simulink library "ddm"  (R2021b)
settings: Solver=VariableStepAuto  StartTime=0.0  StopTime=10.0  RelTol=1e-3
undefined symbols (not defined in the file): ADDM_FrTMTqDev_X_Nm, ADDM_RrTMTqDev_X_Nm, ENUM_ADASACCSTA_ERROR, ENUM_ADASACCSTA_OFF, ENUM_ADASACCSTA_STANDBY, ENUM_ALLOWMOV_ALLOWREADY, ENUM_APS, ENUM_BRKSTA_ERROR, ENUM_BRKSTA_OFF, ENUM_BRKSTA_ON, ENUM_BRKSW_INVALID, ENUM_BRKSW_OFF, ENUM_BRKSW_ON, ENUM_CHGPREACTERRSTA_OBCPRE, ENUM_DCDCFAULTSTA_ANYFAULTLV1, ENUM_DCDCFAULTSTA_ANYFAULTLV2, ENUM_DRIVETRAIN_AWD, ENUM_DRIVETRAIN_FWD, ENUM_DRIVETRAIN_RWD, ENUM_EDUDRTSTA_NORMAL, ENUM_EPBERROR_FAILED, ENUM_EPBSTA_APPLIED, ENUM_EPBSTA_RELEASED, ENUM_ESCAPSSta_APSUNAVAILABLE, ENUM_GEARACTUALPOSN_INVALID, ENUM_GEARACTUALPOSN_P, ENUM_HVBATTREADYPRE_READY, ENUM_HWRESETSTA_HWRESETING, ENUM_MCUWARN_LV0, ENUM_MCUWARN_LV1, ENUM_MCUWARN_LV2, ENUM_MCUWARN_LV3, ENUM_MCUWARN_NOERROR, ENUM_OBCFAULTSTA_ANYFAULT, ENUM_PAS_R2F2, ENUM_PDFAULT_BATTPDFAIL, ENUM_PDFAULT_DCDCDISABLE, ENUM_PDFAULT_MCUDISABLE, ENUM_PDFAULT_MCUDISCHRG, ENUM_POWERSTA_OFF, ENUM_POWERSTA_ON, ENUM_POWERSTA_READY, ENUM_POWERSTA_STANDBY, ENUM_PRESSINDI_LOW, ENUM_PUFAULT_BATTUPFAIL, ENUM_PUFAULT_DCDCENABLEFAIL, ENUM_PUFAULT_PRECHRGCHKFAIL, ENUM_PUFAULT_SAFETYCHKFAIL, ENUM_PWRSTASW_OFF, ENUM_PWRSTASW_OFFA, ENUM_PWRSTASW_OFFCHVCHRG, ENUM_PWRSTASW_OFFCLVCHRG, ENUM_PWRSTASW_ON, ENUM_PWRSTASW_ONHVCHRG, ENUM_PWRSTASW_READY, ENUM_PWRSTASW_STANDBY, ENUM_RAPSErrWarnSta_NORMAL, ENUM_RAPSErrWarnSta_RAPSERRLV1, ENUM_SHIFTCOMMAND_P, ENUM_SHIFTERERRSTA_PBUTTONFAILURE ... (+471)
libraries: hcu_lib x540, simulink x3
(part 15 of 26)

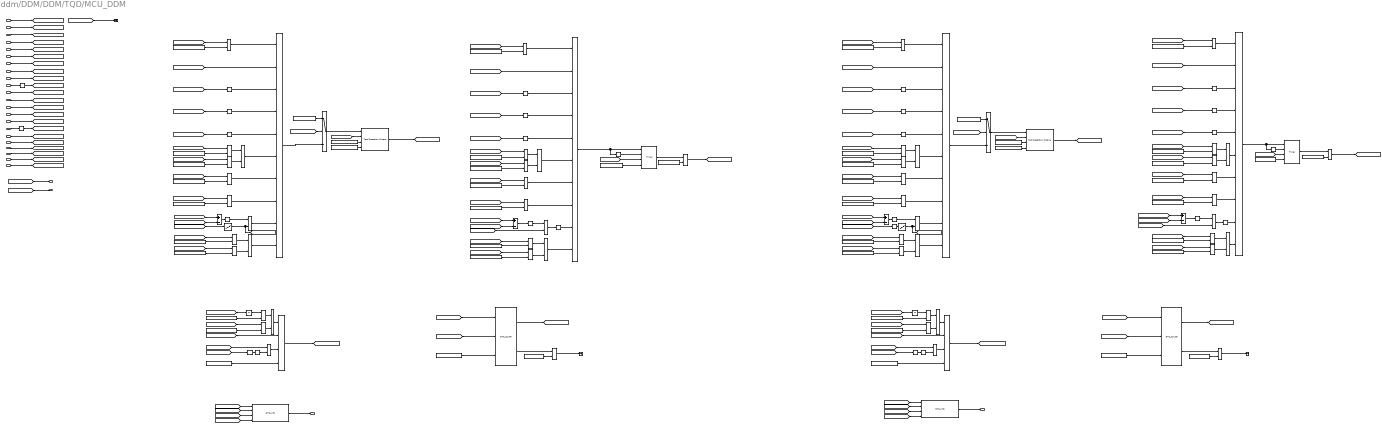
== system ddm/DDM/DDM/TQD/MCU_DDM ==
  note: VINP_FrEDUDrtSta_flg
  note: Front Motor Torque Response Error (FrMCUTqErr)
  note: Test Pass Creteria
  note: Test Dtection Criteria
  note: Test Pass Creteria
  note: Rear Motor Torque Response Error (RrMCUTqErr)
  note: Test Dtection Criteria
  note: Diagnostics and Fault Handling
  note: Release Condition After Decision
  note: Release Condition After Decision
  note: Diagnostics and Fault Handling
  task_time_s : Inport
  VPMM_SysPwrSta_enum : Inport  Port=2
  No_CAN3_BUS_OFF : Inport  Port=3
  VDDM_MCUF1NoComCFS_flg : Inport  Port=4
  VDDM_MCUF1RCErrCFS_flg : Inport  Port=5
  VDDM_MCUF1CSErrCFS_flg : Inport  Port=6
  VINP_VehSpeed_kph : Inport  Port=7
  VINP_FrEDUDrtSta_flg : Inport  Port=8
  VINP_FrEDURealTMTq_Nm : Inport  Port=9
  VTQR_FrTMTqReq_Nm : Inport  Port=10
  VDDM_MCUR1NoComCFS_flg : Inport  Port=11
  VDDM_MCUR1RCErrCFS_flg : Inport  Port=12
  VDDM_MCUR1CSErrCFS_flg : Inport  Port=13
  VINP_RrEDUDrtSta_flg : Inport  Port=14
  VINP_RrEDURealTMTq_Nm : Inport  Port=15
  VTQR_RrTMTqReq_Nm : Inport  Port=16
  VINP_MCUWarnF_enum : Inport  Port=17
  VINP_MCUWarnR_enum : Inport  Port=18
  DTC_clear_request : Inport  Port=19
  VPMM_DrivetrainSelect_enum : Inport  Port=20
  VTQR_FrTqZeroTrans_enum : Inport  Port=21
  VTQR_RrTqZeroTrans_enum : Inport  Port=22
  Abs{,1..3,6} (5 alike) : Abs
  Add{,1..3} (4 alike) : Sum  Inputs=+-
  Constant1 : Constant  Value=ENUM_DRIVETRAIN_FWD
  Constant{3,7,10,31} (4 alike) : Constant  Value=ENUM_TQZEROTRANS_NOZEROTRANS
  Constant{4,11,16,32} (4 alike) : Constant  Value=ENUM_MCUWARN_LV0
  Constant12 : Constant  Value=ENUM_PWRSTASW_STANDBY
  Constant{13,17,19,23,33,44} (6 alike) : Constant  Value=ENUM_PWRSTASW_OFF
  Constant{5,14,21,34} (4 alike) : Constant  Value=ENUM_MCUWARN_NOERROR
  Constant15 : Constant  Value=ENUM_DRIVETRAIN_FWD
  Constant18 : Constant  Value=KDDM_RrMCUTqErrDTC_cnt
  Constant2 : Constant  Value=ENUM_DRIVETRAIN_RWD
  Constant{8,20,26,49} (4 alike) : Constant  Value=ENUM_DRIVETRAIN_AWD
  Constant22 : Constant  Value=ENUM_PWRSTASW_STANDBY
  Constant24 : Constant  Value=FALSE
  Constant{6,25,35,41} (4 alike) : Constant  Value=ENUM_EDUDRTSTA_NORMAL
  Constant28 : Constant  Value=KDDM_RrMCUTqErrDTC_cnt
  Constant29 : Constant  Value=KDDM_TQDDiagnosisOffSW_flg
  Constant30 : Constant  Value=ZERO_INT
  Constant36 : Constant  Value=KDDM_RrMCUTqErrPassTO_s
  Constant37 : Constant  Value=KDDM_RrMCUTqErrDetTO_s
  Constant39 : Constant  Value=KDDM_RrMCUTqErrPassTO_s
  Constant42 : Constant  Value=FALSE
  Constant43 : Constant  Value=KDDM_FrMCUTqErrDTC_cnt
  Constant45 : Constant  Value=KDDM_FrMCUTqErrPassTO_s
  Constant46 : Constant  Value=KDDM_FrMCUTqErrDetTO_s
  Constant51 : Constant  Value=KDDM_TQDDiagnosisOffSW_flg
  Constant52 : Constant  Value=ZERO_INT
  Constant54 : Constant  Value=KDDM_FrMCUTqErrDTC_cnt
  Constant70 : Constant  Value=KDDM_FrMCUTqErrPassTO_s
  Constant9 : Constant  Value=ENUM_DRIVETRAIN_RWD
  DTC_Couter1 : hcu_lib/Basic_Blocks/DTC_Couter
  DTC_Couter3 : hcu_lib/Basic_Blocks/DTC_Couter
  DTC_Info : hcu_lib/Basic_Blocks/DTC_Info
  DTC_Info1 : hcu_lib/Basic_Blocks/DTC_Info
  Delay1 : Delay  DelayLength=1
  Delay2 : Delay  DelayLength=1
  Equal{,1..4,6..7,9..11,14..15,17,20..23,25,28..37} (28 alike) : RelationalOperator  Operator===  OutDataTypeStr=boolean  RndMeth=Simplest
  Equal{5,8,12..13,18,27} (6 alike) : RelationalOperator  OutDataTypeStr=boolean  RndMeth=Simplest
  Equal{16,19,24,26} (4 alike) : RelationalOperator  Operator=~=  OutDataTypeStr=boolean  RndMeth=Simplest
  Logical Operator{1..2,4,16} (4 alike) : Logic  Operator=OR  AllPortsSameDT=off  OutDataTypeStr=boolean
  Logical Operator{3,5,7..10,12..15,17..18,28,34..35,37} (16 alike) : Logic  Operator=NOT  AllPortsSameDT=off  OutDataTypeStr=boolean
  Logical Operator{6,11,27,30} (4 alike) : Logic  Inputs=10  AllPortsSameDT=off  OutDataTypeStr=boolean
  Logical Operator19 : Logic  Operator=OR  Inputs=4  AllPortsSameDT=off  OutDataTypeStr=boolean
  Logical Operator{20..22,43} (4 alike) : Logic  AllPortsSameDT=off  OutDataTypeStr=boolean
  Logical Operator41 : Logic  Operator=OR  Inputs=4  AllPortsSameDT=off  OutDataTypeStr=boolean
  MDDM_FrTMTqDev_Y_Nm : Lookup_n-D  NumberOfTableDimensions=1  BreakpointsForDimension1=ADDM_FrTMTqDev_X_Nm  Table=MDDM_FrTMTqDev_Y_Nm  InternalRulePriority=Speed  RndMeth=Simplest  InputSameDT=on
  MDDM_RrTMTqDev_Y_Nm : Lookup_n-D  NumberOfTableDimensions=1  BreakpointsForDimension1=ADDM_RrTMTqDev_X_Nm  Table=MDDM_RrTMTqDev_Y_Nm  InternalRulePriority=Speed  RndMeth=Simplest  InputSameDT=on
  NOT1 : Logic  Operator=NOT  AllPortsSameDT=off  OutDataTypeStr=boolean
  NOT2 : Logic  Operator=NOT  AllPortsSameDT=off  OutDataTypeStr=boolean
  OR{,1..3} (4 alike) : Logic  Operator=OR  AllPortsSameDT=off  OutDataTypeStr=boolean
  Relational Operator1 : RelationalOperator  Operator=>  OutDataTypeStr=boolean  RndMeth=Simplest
  Relational Operator2 : RelationalOperator  Operator=>  OutDataTypeStr=boolean  RndMeth=Simplest
  Round : Rounding  Operator=round
  Round1 : Rounding  Operator=round
  Switch1 : Switch  Criteria=u2 ~= 0
  Switch6 : Switch  Criteria=u2 ~= 0
  Terminator : Terminator
  Terminator1 : Terminator
  Terminator2 : Terminator
  Test Detection Criteria1 : hcu_lib/Basic_Blocks/Test Detection Criteria
  Test Detection Criteria2 : hcu_lib/Basic_Blocks/Test Detection Criteria
  Timer1 : hcu_lib/Basic_Blocks/Timer
  Timer2 : hcu_lib/Basic_Blocks/Timer
  Unit Delay1 : UnitDelay  SampleTime=-1  HasFrameUpgradeWarning=on
  Unit Delay5 : UnitDelay  SampleTime=-1  HasFrameUpgradeWarning=on
  VDDM_FrMCUTqErrDTC_raw32 : Outport
  VDDM_RrMCUTqErrDTC_raw32 : Outport  Port=2
  VDDM_FrMCUTqErrCFS_flg : Outport  Port=3
  VDDM_RrMCUTqErrCFS_flg : Outport  Port=4
  wires:
  Equal26/1 -> Logical Operator30/1
  Constant44/1 -> Equal26/2
  [VPMM_SysPwrSta_enum] -> Equal26/1
  [No_CAN_BUS_OFF] -> Logical Operator30/2
  Constant4/1 -> Equal6/2
  Constant5/1 -> Equal7/2
  Equal6/1 -> Logical Operator1/1
  Equal7/1 -> Logical Operator1/2
  Logical Operator1/1 -> Logical Operator30/6
  [VINP_FrEDUDrtSta_flg] -> Equal10/1
  Constant6/1 -> Equal10/2
  Equal10/1 -> Logical Operator30/7
  Equal2/1 -> Logical Operator30/8
  [VDDM_MCUF1CSErrCFS_flg] -> Logical Operator10/1
  [VDDM_MCUF1RCErrCFS_flg] -> Logical Operator9/1
  Logical Operator9/1 -> Logical Operator30/4
  [VDDM_MCUF1NoComCFS_flg] -> Logical Operator7/1
  Logical Operator7/1 -> Logical Operator30/3
  Logical Operator10/1 -> Logical Operator30/5
  [VDDM_MCUR1CSErrCFS_flg] -> Logical Operator17/1
  Equal33/1 -> Logical Operator16/1
  [VINP_MCUWarnR_enum] -> Equal33/1
  [VINP_MCUWarnR_enum] -> Equal34/1
  Logical Operator17/1 -> Logical Operator27/5
  Equal34/1 -> Logical Operator16/2
  [VDDM_MCUR1NoComCFS_flg] -> Logical Operator35/1
  Constant33/1 -> Equal24/2
  Equal23/1 -> Logical Operator27/8
  Equal9/1 -> Logical Operator27/7
  [VDDM_MCUR1RCErrCFS_flg] -> Logical Operator37/1
  Constant35/1 -> Equal9/2
  Logical Operator35/1 -> Logical Operator27/3
  Constant32/1 -> Equal33/2
  [VINP_RrEDUDrtSta_flg] -> Equal9/1
  Constant34/1 -> Equal34/2
  [No_CAN_BUS_OFF] -> Logical Operator27/2
  Logical Operator16/1 -> Logical Operator27/6
  Equal24/1 -> Logical Operator27/1
  [VPMM_SysPwrSta_enum] -> Equal24/1
  Logical Operator37/1 -> Logical Operator27/4
  Logical Operator11/1 -> Logical Operator34/1, Timer1/1
  [task_time_s] -> Test Detection Criteria1/2
  [task_time_s] -> Timer1/3
  Constant42/1 -> Switch6/1
  Test Detection Criteria1/1 -> [VDDM_FrMCUTqErrDet_flg]  "VDDM_FrMCUTqErrDet_flg"
  Logical Operator34/1 -> Timer1/2
  Timer1/1 -> Equal27/1
  Constant43/1 -> Test Detection Criteria1/3
  Switch6/1 -> Test Detection Criteria1/1
  Equal27/1 -> [VDDM_FrMCUTqErrPass_flg]  "VDDM_FrMCUTqErrPass_flg"
  Logical Operator30/1 -> Switch6/3
  Constant46/1 -> Test Detection Criteria1/4
  Constant70/1 -> Timer1/4
  Constant45/1 -> Equal27/2
  [VDDM_FrMCUTqErrCFSRls_flg] -> Switch6/2
  [VDDM_FrMCUTqErrDet_flg] -> DTC_Info/1
  DTC_Info/1 -> VDDM_FrMCUTqErrDTC_raw32/1  "VDDM_FrMCUTqErrDTC_raw32"
  [DTC_clear_request] -> DTC_Info/4
  [VDDM_FrMCUTqErrCFS_flg] -> DTC_Info/3
  [VDDM_FrMCUTqErrPass_flg] -> DTC_Info/2
  [VDDM_RrMCUTqErrCFSRls_flg] -> Switch1/2
  Test Detection Criteria2/1 -> [VDDM_RrMCUTqErrDet_flg]  "VDDM_RrMCUTqErrDet_flg"
  [VDDM_RrMCUTqErrDet_flg] -> DTC_Info1/1
  DTC_Info1/1 -> VDDM_RrMCUTqErrDTC_raw32/1  "VDDM_RrMCUTqErrDTC_raw32"
  [DTC_clear_request] -> DTC_Info1/4
  Equal5/1 -> [VDDM_RrMCUTqErrPass_flg]  "VDDM_RrMCUTqErrPass_flg"
  [VDDM_RrMCUTqErrCFS_flg] -> DTC_Info1/3
  Constant39/1 -> Timer2/4
  Constant24/1 -> Switch1/1
  [task_time_s] -> Timer2/3
  Timer2/1 -> Equal5/1
  [VDDM_RrMCUTqErrPass_flg] -> DTC_Info1/2
  [task_time_s] -> Test Detection Criteria2/2
  Constant28/1 -> Test Detection Criteria2/3
  Logical Operator27/1 -> Switch1/3
  Constant37/1 -> Test Detection Criteria2/4
  Switch1/1 -> Test Detection Criteria2/1
  Logical Operator28/1 -> Timer2/2
  Constant36/1 -> Equal5/2
  Logical Operator6/1 -> Logical Operator28/1, Timer2/1
  task_time_s/1 -> [task_time_s]
  VPMM_SysPwrSta_enum/1 -> [VPMM_SysPwrSta_enum]
  No_CAN3_BUS_OFF/1 -> [No_CAN_BUS_OFF]
  VDDM_MCUF1NoComCFS_flg/1 -> [VDDM_MCUF1NoComCFS_flg]
  VDDM_MCUF1RCErrCFS_flg/1 -> [VDDM_MCUF1RCErrCFS_flg]
  VDDM_MCUF1CSErrCFS_flg/1 -> [VDDM_MCUF1CSErrCFS_flg]
  VINP_FrEDUDrtSta_flg/1 -> [VINP_FrEDUDrtSta_flg]
  VINP_VehSpeed_kph/1 -> [VINP_VehSpeed_kph]
  VTQR_FrTMTqReq_Nm/1 -> Round1/1
  VDDM_MCUR1NoComCFS_flg/1 -> [VDDM_MCUR1NoComCFS_flg]
  VDDM_MCUR1RCErrCFS_flg/1 -> [VDDM_MCUR1RCErrCFS_flg]
  VDDM_MCUR1CSErrCFS_flg/1 -> [VDDM_MCUR1CSErrCFS_flg]
  VINP_RrEDUDrtSta_flg/1 -> [VINP_RrEDUDrtSta_flg]
  VTQR_RrTMTqReq_Nm/1 -> Round/1
  DTC_clear_request/1 -> [DTC_clear_request]
  [VINP_MCUWarnF_enum] -> Equal6/1
  [VINP_MCUWarnF_enum] -> Equal7/1
  Round/1 -> [VTQR_RrTMTqReq_Nm]
  VINP_RrEDURealTMTq_Nm/1 -> [VINP_RrEDURealTMTq_Nm]
  Round1/1 -> [VTQR_FrTMTqReq_Nm]
  VINP_FrEDURealTMTq_Nm/1 -> [VINP_FrEDURealTMTq_Nm]
  OR/1 -> Logical Operator30/10
  Constant15/1 -> Equal/2
  Constant49/1 -> Equal25/2
  [VPMM_DrivetrainSelect_enum] -> Equal25/1
  [VPMM_DrivetrainSelect_enum] -> Equal/1
  Equal25/1 -> OR/2
  Equal/1 -> OR/1
  MDDM_FrTMTqDev_Y_Nm/1 -> [VDDM_FrTMTqDev_Nm], Equal12/2  "VDDM_FrTMTqDev_Nm"
  Abs/1 -> Equal12/1  "VDDM_FrTMTqDiffAbs_Nm"
  Add/1 -> Abs/1
  [VINP_FrEDURealTMTq_Nm] -> Add/1
  Equal12/1 -> Logical Operator30/9  "VDDM_FrTMTqDiffGTDev_flg"
  [VTQR_FrTMTqReq_Nm] -> MDDM_FrTMTqDev_Y_Nm/1
  [VTQR_FrTMTqReq_Nm] -> Add/2
  VPMM_DrivetrainSelect_enum/1 -> [VPMM_DrivetrainSelect_enum]
  [VPMM_DrivetrainSelect_enum] -> Equal1/1
  Equal15/1 -> OR1/2
  Constant1/1 -> Equal1/2
  Add1/1 -> Abs1/1
  [No_CAN_BUS_OFF] -> Logical Operator11/2
  Equal14/1 -> Logical Operator11/8
  Equal11/1 -> Logical Operator11/7
  Equal28/1 -> Logical Operator2/1
  Logical Operator14/1 -> Logical Operator11/4
  Logical Operator3/1 -> Logical Operator11/5
  Logical Operator2/1 -> Logical Operator11/6
  Equal1/1 -> OR1/1
  [VPMM_SysPwrSta_enum] -> Equal16/1
  Constant21/1 -> Equal29/2
  Constant17/1 -> Equal16/2
  Constant20/1 -> Equal15/2
  [VPMM_DrivetrainSelect_enum] -> Equal15/1
  Equal16/1 -> Logical Operator11/1
  Logical Operator13/1 -> Logical Operator11/3
  Constant41/1 -> Equal11/2
  [VDDM_MCUF1NoComCFS_flg] -> Logical Operator13/1
  [VDDM_MCUF1RCErrCFS_flg] -> Logical Operator14/1
  [VINP_MCUWarnF_enum] -> Equal29/1
  [VINP_FrEDUDrtSta_flg] -> Equal11/1
  Constant16/1 -> Equal28/2
  Abs1/1 -> Equal13/1
  [VINP_MCUWarnF_enum] -> Equal28/1
  Equal29/1 -> Logical Operator2/2
  [VINP_FrEDURealTMTq_Nm] -> Add1/1
  [VTQR_FrTMTqReq_Nm] -> Add1/2
  OR1/1 -> Logical Operator11/10
  [VDDM_MCUF1CSErrCFS_flg] -> Logical Operator3/1
  Equal13/1 -> Logical Operator15/1
  Logical Operator15/1 -> Logical Operator11/9
  Constant52/1 -> Relational Operator2/2
  [VDDM_FrMCUTqErrDet_flg] -> DTC_Couter3/1
  DTC_Couter3/2 -> Relational Operator2/1  "VDDM_FrMCUTqErrDTC_cnt"
  [VDDM_FrMCUTqErrCFSRls_flg] -> DTC_Couter3/2
  Logical Operator41/1 -> [VDDM_FrMCUTqErrCFSRls_flg]  "VDDM_FrMCUTqErrCFSRls_flg"
  DTC_Couter3/1 -> [VDDM_FrMCUTqErrCFS_flg]  "VDDM_FrMCUTqErrCFS_flg"
  Constant54/1 -> DTC_Couter3/3
  Logical Operator43/1 -> Logical Operator41/3
  [VDDM_FrMCUTqErrPass_flg] -> Logical Operator43/1
  Relational Operator2/1 -> Terminator/1  "VDDM_FrMCUTqErrDFS_flg"
  Logical Operator20/1 -> Logical Operator41/1
  NOT1/1 -> Logical Operator43/2
  [DTC_clear_request] -> Logical Operator41/2
  Constant51/1 -> Logical Operator41/4
  [VDDM_FrMCUTqErrCFS_flg] -> Delay1/1
  Delay1/1 -> NOT1/1
  [VTQR_RrTMTqReq_Nm] -> Abs6/1
  Abs2/1 -> Equal18/1  "VDDM_RrTMTqDiffAbs_Nm"
  Abs6/1 -> MDDM_RrTMTqDev_Y_Nm/1
  OR2/1 -> Logical Operator27/10
  [VPMM_DrivetrainSelect_enum] -> Equal3/1
  Constant8/1 -> Equal4/2
  Constant2/1 -> Equal3/2
  Equal3/1 -> OR2/1
  Equal4/1 -> OR2/2
  Add2/1 -> Abs2/1
  Equal18/1 -> Logical Operator27/9  "VDDM_RrTMTqDiffGTDev_flg"
  [VTQR_RrTMTqReq_Nm] -> Add2/2
  [VPMM_DrivetrainSelect_enum] -> Equal4/1
  [VINP_RrEDURealTMTq_Nm] -> Add2/1
  MDDM_RrTMTqDev_Y_Nm/1 -> [VDDM_RrTMTqDev_Nm], Equal18/2  "VDDM_RrTMTqDev_Nm"
  Add3/1 -> Abs3/1
  [VPMM_DrivetrainSelect_enum] -> Equal20/1
  Logical Operator4/1 -> Logical Operator6/6
  Logical Operator12/1 -> Logical Operator6/4
  [No_CAN_BUS_OFF] -> Logical Operator6/2
  Constant14/1 -> Equal22/2
  Logical Operator8/1 -> Logical Operator6/3
  Constant25/1 -> Equal37/2
  [VDDM_MCUR1NoComCFS_flg] -> Logical Operator8/1
  Equal37/1 -> Logical Operator6/7
  Constant13/1 -> Equal19/2
  Equal22/1 -> Logical Operator4/2
  Equal21/1 -> Logical Operator4/1
  [VDDM_MCUR1CSErrCFS_flg] -> Logical Operator5/1
  [VINP_RrEDURealTMTq_Nm] -> Add3/1
  Equal19/1 -> Logical Operator6/1
  [VPMM_SysPwrSta_enum] -> Equal19/1
  [VINP_MCUWarnR_enum] -> Equal22/1
  Logical Operator5/1 -> Logical Operator6/5
  [VINP_MCUWarnR_enum] -> Equal21/1
  Abs3/1 -> Equal8/1
  Equal36/1 -> OR3/2
  [VPMM_DrivetrainSelect_enum] -> Equal36/1
  [VINP_RrEDUDrtSta_flg] -> Equal37/1
  Equal20/1 -> OR3/1
  [VDDM_MCUR1RCErrCFS_flg] -> Logical Operator12/1
  OR3/1 -> Logical Operator6/10
  [VTQR_RrTMTqReq_Nm] -> Add3/2
  Constant9/1 -> Equal20/2
  Constant11/1 -> Equal21/2
  Constant26/1 -> Equal36/2
  Equal8/1 -> Logical Operator18/1
  Logical Operator18/1 -> Logical Operator6/9
  Constant30/1 -> Relational Operator1/2
  DTC_Couter1/2 -> Relational Operator1/1  "VDDM_RrMCUTqErrDTC_cnt"
  [DTC_clear_request] -> Logical Operator19/2
  Constant18/1 -> DTC_Couter1/3
  Constant29/1 -> Logical Operator19/4
  NOT2/1 -> Logical Operator22/2
  Delay2/1 -> NOT2/1
  [VDDM_RrMCUTqErrCFSRls_flg] -> DTC_Couter1/2
  DTC_Couter1/1 -> [VDDM_RrMCUTqErrCFS_flg]  "VDDM_RrMCUTqErrCFS_flg"
  Logical Operator21/1 -> Logical Operator19/1
  [VDDM_RrMCUTqErrDet_flg] -> DTC_Couter1/1
  [VDDM_RrMCUTqErrCFS_flg] -> Delay2/1
  Relational Operator1/1 -> Terminator1/1  "VDDM_RrMCUTqErrDFS_flg"
  [VDDM_RrMCUTqErrPass_flg] -> Logical Operator22/1
  Logical Operator22/1 -> Logical Operator19/3
  Logical Operator19/1 -> [VDDM_RrMCUTqErrCFSRls_flg]  "VDDM_RrMCUTqErrCFSRls_flg"
  [VDDM_FrTMTqDev_Nm] -> Equal13/2
  [VDDM_RrTMTqDev_Nm] -> Equal8/2
  [VDDM_FrMCUTqErrCFS_flg] -> VDDM_FrMCUTqErrCFS_flg/1
  [VDDM_RrMCUTqErrCFS_flg] -> VDDM_RrMCUTqErrCFS_flg/1
  Constant19/1 -> Equal31/2
  Constant12/1 -> Equal30/2
  [VPMM_SysPwrSta_enum] -> Equal30/1
  Equal31/1 -> Logical Operator20/1
  Unit Delay5/1 -> Equal31/1
  Equal30/1 -> Logical Operator20/2
  [VPMM_SysPwrSta_enum] -> Unit Delay5/1
  Constant23/1 -> Equal35/2
  Constant22/1 -> Equal32/2
  [VPMM_SysPwrSta_enum] -> Equal32/1
  Equal35/1 -> Logical Operator21/1
  Unit Delay1/1 -> Equal35/1
  Equal32/1 -> Logical Operator21/2
  [VPMM_SysPwrSta_enum] -> Unit Delay1/1
  VINP_MCUWarnF_enum/1 -> [VINP_MCUWarnF_enum]
  VINP_MCUWarnR_enum/1 -> [VINP_MCUWarnR_enum]
  Constant3/1 -> Equal2/2
  [VTQR_FrTqZeroTrans_enum] -> Equal2/1
  Constant7/1 -> Equal14/2
  [VTQR_FrTqZeroTrans_enum] -> Equal14/1
  VTQR_RrTqZeroTrans_enum/1 -> [VTQR_RrTqZeroTrans_enum]
  VTQR_FrTqZeroTrans_enum/1 -> [VTQR_FrTqZeroTrans_enum]
  [VTQR_RrTqZeroTrans_enum] -> Equal23/1
  Constant31/1 -> Equal23/2
  Constant10/1 -> Equal17/2
  Equal17/1 -> Logical Operator6/8
  [VTQR_RrTqZeroTrans_enum] -> Equal17/1
  [VINP_VehSpeed_kph] -> Terminator2/1

== system ddm/DDM/DDM/TQD/Regen_fail_DDM ==
  note: Diagnostics and Fault Handling
  note: Test Dtection Criteria
  note: Test Pass Creteria
  note: Regen Fail
  note: Release Condition After Decision
  task_time_s : Inport
  VPMM_SysPwrSta_enum : Inport  Port=2
  VDDM_LimpHomeAct_flg : Inport  Port=3
  DTC_clear_request : Inport  Port=4
  Constant1 : Constant  Value=KDDM_RegenErrDTC_cnt
  Constant17 : Constant  Value=ENUM_PWRSTASW_READY
  Constant2 : Constant  Value=FALSE
  Constant20 : Constant  Value=KDDM_RegenErrDTC_cnt
  Constant21 : Constant  Value=KDDM_RegenErrPassTO_s
  Constant22 : Constant  Value=KDDM_RegenErrDetTO_s
  Constant26 : Constant  Value=ENUM_PWRSTASW_STANDBY
  Constant3 : Constant  Value=ENUM_PWRSTASW_READY
  Constant44 : Constant  Value=KDDM_TQDDiagnosisOffSW_flg
  Constant45 : Constant  Value=ZERO_INT
  Constant48 : Constant  Value=ENUM_PWRSTASW_OFF
  Constant70 : Constant  Value=KDDM_RegenErrPassTO_s
  DTC_Couter4 : hcu_lib/Basic_Blocks/DTC_Couter
  DTC_Info : hcu_lib/Basic_Blocks/DTC_Info
  Data Type Conversion : DataTypeConversion  OutDataTypeStr=boolean
  Data Type Conversion1 : DataTypeConversion  OutDataTypeStr=boolean
  Delay : Delay  DelayLength=1
  Equal{1,6,17..18} (4 alike) : RelationalOperator  Operator===  OutDataTypeStr=boolean  RndMeth=Simplest
  Equal7 : RelationalOperator  OutDataTypeStr=boolean  RndMeth=Simplest
  Logical Operator1 : Logic  Operator=NOT  AllPortsSameDT=off  OutDataTypeStr=boolean
  Logical Operator10 : Logic  AllPortsSameDT=off  OutDataTypeStr=boolean
  Logical Operator48 : Logic  Operator=OR  Inputs=4  AllPortsSameDT=off  OutDataTypeStr=boolean
  Logical Operator5 : Logic  AllPortsSameDT=off  OutDataTypeStr=boolean
  Logical Operator50 : Logic  AllPortsSameDT=off  OutDataTypeStr=boolean
  Relational Operator2 : RelationalOperator  Operator=>  OutDataTypeStr=boolean  RndMeth=Simplest
  Switch6 : Switch  Criteria=u2 ~= 0
  Terminator : Terminator
  Test Detection Criteria1 : hcu_lib/Basic_Blocks/Test Detection Criteria
  Timer2 : hcu_lib/Basic_Blocks/Timer
  Unit Delay6 : UnitDelay  SampleTime=-1  HasFrameUpgradeWarning=on
  VDDM_RegenErrDTC_raw32 : Outport
  VDDM_RegenErrCFS_flg : Outport  Port=2
  wires:
  Constant17/1 -> Equal6/2
  Timer2/1 -> Equal7/1
  Constant22/1 -> Test Detection Criteria1/4
  Equal7/1 -> [VDDM_RegenErrPass_flg]  "VDDM_RegenErrPass_flg"
  [task_time_s] -> Timer2/3
  [VDDM_RegenErrDet_flg] -> DTC_Couter4/1
  Constant20/1 -> Test Detection Criteria1/3
  [DTC_clear_request] -> DTC_Info/4
  Logical Operator48/1 -> [VDDM_RegenErrCFSRls_flg]  "VDDM_RegenErrCFSRls_flg"
  [VPMM_SysPwrSta_enum] -> Equal6/1
  DTC_Info/1 -> VDDM_RegenErrDTC_raw32/1  "VDDM_RegenErrDTC_raw32"
  Equal18/1 -> Logical Operator50/1
  Test Detection Criteria1/1 -> [VDDM_RegenErrDet_flg]  "VDDM_RegenErrDet_flg"
  [VDDM_RegenErrCFS_flg] -> DTC_Info/3
  Logical Operator10/1 -> Switch6/3
  [VDDM_RegenErrPass_flg] -> DTC_Info/2
  [VDDM_RegenErrDet_flg] -> DTC_Info/1
  Switch6/1 -> Test Detection Criteria1/1
  [VDDM_RegenErrCFSRls_flg] -> Switch6/2
  Constant2/1 -> Switch6/1
  DTC_Couter4/1 -> [VDDM_RegenErrCFS_flg]  "VDDM_RegenErrCFS_flg"
  [VDDM_RegenErrCFSRls_flg] -> DTC_Couter4/2
  [VDDM_RegenErrPass_flg] -> Logical Operator48/3
  Constant21/1 -> Equal7/2
  [VPMM_SysPwrSta_enum] -> Equal17/1
  Constant44/1 -> Logical Operator48/4
  Constant70/1 -> Timer2/4
  Constant26/1 -> Equal17/2
  Logical Operator50/1 -> Logical Operator48/1
  Constant45/1 -> Relational Operator2/2
  Constant1/1 -> DTC_Couter4/3
  Relational Operator2/1 -> Terminator/1  "VDDM_RegenErrDFS_flg"
  Equal17/1 -> Logical Operator50/2
  Logical Operator5/1 -> Timer2/2, Logical Operator1/1
  Unit Delay6/1 -> Equal18/1
  Constant48/1 -> Equal18/2
  [VPMM_SysPwrSta_enum] -> Unit Delay6/1
  DTC_Couter4/2 -> Relational Operator2/1  "VDDM_RegenErrDTC_cnt"
  [task_time_s] -> Test Detection Criteria1/2
  [DTC_clear_request] -> Logical Operator48/2
  Logical Operator1/1 -> Timer2/1
  Equal6/1 -> Logical Operator10/2
  [VDDM_LimpHomeAct_flg] -> Data Type Conversion/1
  [VPMM_SysPwrSta_enum] -> Equal1/1
  Constant3/1 -> Equal1/2
  Equal1/1 -> Logical Operator5/2
  VPMM_SysPwrSta_enum/1 -> [VPMM_SysPwrSta_enum]
  VDDM_LimpHomeAct_flg/1 -> Delay/1
  DTC_clear_request/1 -> [DTC_clear_request]
  [VDDM_RegenErrCFS_flg] -> VDDM_RegenErrCFS_flg/1
  task_time_s/1 -> [task_time_s]
  Data Type Conversion/1 -> Logical Operator10/1
  [VDDM_LimpHomeAct_flg] -> Data Type Conversion1/1
  Data Type Conversion1/1 -> Logical Operator5/1
  Delay/1 -> [VDDM_LimpHomeAct_flg]

== system ddm/DDM/DDM/TQD/Shifter1_DDM ==
  note: Release Condition After Decision
  note: Diagnostics and Fault Handling
  note: Diagnostics and Fault Handling
  note: Release Condition After Decision
  note: Release Condition After Decision
  note: Diagnostics and Fault Handling
  note: Shifter1 Rolling Count Error (Shifter1CSErr)
  note: Shifter1 Rolling Count Error (Shifter1RCErr)
  note: Shifter1 Lost Comm (Shifter1NoCom)
  task_time_s : Inport
  VPMM_SysPwrSta_enum : Inport  Port=2
  No_CAN3_BUS_OFF : Inport  Port=3
  VDDM_Shifter1NoCom_flg : Inport  Port=4
  VDDM_Shifter1RCErr_flg : Inport  Port=5
  VDDM_Shifter1CSErr_flg : Inport  Port=6
  DTC_clear_request : Inport  Port=7
  VINP_ShifterHandleCmd_enum : Inport  Port=8
  Constant1 : Constant  Value=KDDM_Shifter1NoComDTC_cnt
  Constant10 : Constant  Value=KDDM_Shifter1CSErrDTC_cnt
  Constant{3,11,16..17,19,24,31,36,48} (9 alike) : Constant  Value=ENUM_PWRSTASW_OFF
  Constant12 : Constant  Value=FALSE
  Constant13 : Constant  Value=KDDM_Shifter1RCErrDTC_cnt
  Constant14 : Constant  Value=KDDM_Shifter1RCErrPassTO_s
  Constant15 : Constant  Value=ZERO_INT
  Constant18 : Constant  Value=KDDM_Shifter1RCErrDetTO_s
  Constant2 : Constant  Value=FALSE
  Constant20 : Constant  Value=KDDM_Shifter1NoComDTC_cnt
  Constant21 : Constant  Value=KDDM_Shifter1NoComPassTO_s
  Constant22 : Constant  Value=KDDM_Shifter1NoComDetTO_s
  Constant23 : Constant  Value=ENUM_SHIFTCOMMAND_P
  Constant25 : Constant  Value=KDDM_TQDDiagnosisOffSW_flg
  Constant26 : Constant  Value=ENUM_PWRSTASW_STANDBY
  Constant27 : Constant  Value=KDDM_Shifter1RCErrPassTO_s
  Constant32 : Constant  Value=FALSE
  Constant33 : Constant  Value=KDDM_Shifter1CSErrDTC_cnt
  Constant34 : Constant  Value=KDDM_Shifter1CSErrPassTO_s
  Constant35 : Constant  Value=KDDM_Shifter1CSErrDetTO_s
  Constant4 : Constant  Value=KDDM_Shifter1RCErrDTC_cnt
  Constant41 : Constant  Value=KDDM_Shifter1CSErrPassTO_s
  Constant42 : Constant  Value=ENUM_SHIFTCOMMAND_P
  Constant44 : Constant  Value=KDDM_TQDDiagnosisOffSW_flg
  Constant45 : Constant  Value=ZERO_INT
  Constant5 : Constant  Value=ENUM_SHIFTCOMMAND_P
  Constant6 : Constant  Value=ENUM_PWRSTASW_STANDBY
  Constant7 : Constant  Value=KDDM_TQDDiagnosisOffSW_flg
  Constant70 : Constant  Value=KDDM_Shifter1NoComPassTO_s
  Constant8 : Constant  Value=ZERO_INT
  Constant9 : Constant  Value=ENUM_PWRSTASW_STANDBY
  DTC_Couter1 : hcu_lib/Basic_Blocks/DTC_Couter
  DTC_Couter2 : hcu_lib/Basic_Blocks/DTC_Couter
  DTC_Couter4 : hcu_lib/Basic_Blocks/DTC_Couter
  DTC_Info : hcu_lib/Basic_Blocks/DTC_Info
  DTC_Info1 : hcu_lib/Basic_Blocks/DTC_Info
  DTC_Info2 : hcu_lib/Basic_Blocks/DTC_Info
  Equal{,1,3,10..11,16..19} (9 alike) : RelationalOperator  Operator===  OutDataTypeStr=boolean  RndMeth=Simplest
  Equal{2,4..6,13..14} (6 alike) : RelationalOperator  Operator=~=  OutDataTypeStr=boolean  RndMeth=Simplest
  Equal15 : RelationalOperator  OutDataTypeStr=boolean  RndMeth=Simplest
  Equal7 : RelationalOperator  OutDataTypeStr=boolean  RndMeth=Simplest
  Equal8 : RelationalOperator  OutDataTypeStr=boolean  RndMeth=Simplest
  Logical Operator : Logic  Operator=OR  Inputs=3  AllPortsSameDT=off  OutDataTypeStr=boolean
  Logical Operator1 : Logic  Operator=OR  Inputs=4  AllPortsSameDT=off  OutDataTypeStr=boolean
  Logical Operator10 : Logic  Inputs=3  AllPortsSameDT=off  OutDataTypeStr=boolean
  Logical Operator{2,5,8,11,50..51} (6 alike) : Logic  AllPortsSameDT=off  OutDataTypeStr=boolean
  Logical Operator{6,9,12,14,20,24,28,30,34,38} (10 alike) : Logic  Operator=NOT  AllPortsSameDT=off  OutDataTypeStr=boolean
  Logical Operator{4,22,26,36} (4 alike) : Logic  Inputs=4  AllPortsSameDT=off  OutDataTypeStr=boolean
  Logical Operator3 : Logic  Operator=OR  Inputs=4  AllPortsSameDT=off  OutDataTypeStr=boolean
  Logical Operator48 : Logic  Operator=OR  Inputs=4  AllPortsSameDT=off  OutDataTypeStr=boolean
  Logical Operator7 : Logic  Inputs=3  AllPortsSameDT=off  OutDataTypeStr=boolean
  Relational Operator1 : RelationalOperator  Operator=>  OutDataTypeStr=boolean  RndMeth=Simplest
  Relational Operator2 : RelationalOperator  Operator=>  OutDataTypeStr=boolean  RndMeth=Simplest
  Relational Operator3 : RelationalOperator  Operator=>  OutDataTypeStr=boolean  RndMeth=Simplest
  Switch1 : Switch  Criteria=u2 ~= 0
  Switch2 : Switch  Criteria=u2 ~= 0
  Switch6 : Switch  Criteria=u2 ~= 0
  Terminator : Terminator
  Terminator1 : Terminator
  Terminator2 : Terminator
  Test Detection Criteria1 : hcu_lib/Basic_Blocks/Test Detection Criteria
  Test Detection Criteria2 : hcu_lib/Basic_Blocks/Test Detection Criteria
  Test Detection Criteria3 : hcu_lib/Basic_Blocks/Test Detection Criteria
  Timer1 : hcu_lib/Basic_Blocks/Timer
  Timer2 : hcu_lib/Basic_Blocks/Timer
  Timer3 : hcu_lib/Basic_Blocks/Timer
  Unit Delay1 : UnitDelay  SampleTime=-1  HasFrameUpgradeWarning=on
  Unit Delay2 : UnitDelay  SampleTime=-1  HasFrameUpgradeWarning=on
  Unit Delay6 : UnitDelay  SampleTime=-1  HasFrameUpgradeWarning=on
  VDDM_Shifter1NoComDTC_raw32 : Outport
  VDDM_Shifter1RCErrDTC_raw32 : Outport  Port=2
  VDDM_Shifter1CSErrDTC_raw32 : Outport  Port=3
  VDDM_Shifter1NoComCFS_flg : Outport  Port=4
  VDDM_Shifter1RCErrCFS_flg : Outport  Port=5
  VDDM_Shifter1CSErrCFS_flg : Outport  Port=6
  VDDM_Shifter1Err_flg : Outport  Port=7
  wires:
  [VPMM_SysPwrSta_enum] -> Equal3/1
  DTC_Couter2/2 -> Relational Operator3/1  "VDDM_Shifter1CSErrDTC_cnt"
  Equal1/1 -> Logical Operator5/2
  [VINP_ShifterHandleCmd_enum] -> Equal1/1
  Logical Operator3/1 -> [VDDM_Shifter1CSErrCFSRls_flg]  "VDDM_Shifter1CSErrCFSRls_flg"
  Constant23/1 -> Equal1/2
  Constant24/1 -> Equal19/2
  Constant8/1 -> Relational Operator3/2
  Logical Operator5/1 -> Logical Operator3/3
  Equal19/1 -> Logical Operator8/1
  Unit Delay1/1 -> Equal19/1
  Constant25/1 -> Logical Operator3/4
  [VDDM_Shifter1CSErrPass_flg] -> Logical Operator5/1
  [VDDM_Shifter1CSErrDet_flg] -> DTC_Couter2/1
  DTC_Couter2/1 -> [VDDM_Shifter1CSErrCFS_flg]  "VDDM_Shifter1CSErrCFS_flg"
  Constant10/1 -> DTC_Couter2/3
  [VDDM_Shifter1CSErrCFSRls_flg] -> DTC_Couter2/2
  [DTC_clear_request] -> Logical Operator3/2
  Relational Operator3/1 -> Terminator2/1  "VDDM_Shifter1CSErrDFS_flg"
  Constant9/1 -> Equal3/2
  Logical Operator8/1 -> Logical Operator3/1
  [VPMM_SysPwrSta_enum] -> Unit Delay1/1
  Equal3/1 -> Logical Operator8/2
  Equal11/1 -> Logical Operator2/2
  DTC_Couter1/1 -> [VDDM_Shifter1RCErrCFS_flg]  "VDDM_Shifter1RCErrCFS_flg"
  [DTC_clear_request] -> Logical Operator1/2
  Logical Operator2/1 -> Logical Operator1/1
  [VPMM_SysPwrSta_enum] -> Unit Delay2/1
  Constant6/1 -> Equal11/2
  Relational Operator1/1 -> Terminator1/1  "VDDM_Shifter1RCErrDFS_flg"
  DTC_Couter1/2 -> Relational Operator1/1  "VDDM_Shifter1RCErrDTC_cnt"
  [VDDM_Shifter1RCErrCFSRls_flg] -> DTC_Couter1/2
  [VINP_ShifterHandleCmd_enum] -> Equal10/1
  Constant5/1 -> Equal10/2
  Equal10/1 -> Logical Operator11/2
  [VDDM_Shifter1RCErrPass_flg] -> Logical Operator11/1
  [VDDM_Shifter1RCErrDet_flg] -> DTC_Couter1/1
  Logical Operator11/1 -> Logical Operator1/3
  Constant15/1 -> Relational Operator1/2
  [VPMM_SysPwrSta_enum] -> Equal11/1
  Equal16/1 -> Logical Operator2/1
  Constant7/1 -> Logical Operator1/4
  Logical Operator1/1 -> [VDDM_Shifter1RCErrCFSRls_flg]  "VDDM_Shifter1RCErrCFSRls_flg"
  Constant16/1 -> Equal16/2
  Unit Delay2/1 -> Equal16/1
  Constant4/1 -> DTC_Couter1/3
  Equal/1 -> Logical Operator51/2
  Constant42/1 -> Equal/2
  VINP_ShifterHandleCmd_enum/1 -> [VINP_ShifterHandleCmd_enum]
  Constant48/1 -> Equal18/2
  Unit Delay6/1 -> Equal18/1
  DTC_Couter4/2 -> Relational Operator2/1  "VDDM_Shifter1NoComDTC_cnt"
  [DTC_clear_request] -> Logical Operator48/2
  Constant26/1 -> Equal17/2
  Logical Operator50/1 -> Logical Operator48/1
  [VPMM_SysPwrSta_enum] -> Unit Delay6/1
  Equal17/1 -> Logical Operator50/2
  Relational Operator2/1 -> Terminator/1  "VDDM_Shifter1NoComDFS_flg"
  Constant44/1 -> Logical Operator48/4
  [VPMM_SysPwrSta_enum] -> Equal17/1
  Equal18/1 -> Logical Operator50/1
  Constant1/1 -> DTC_Couter4/3
  [VDDM_Shifter1NoComDet_flg] -> DTC_Couter4/1
  [VDDM_Shifter1NoComPass_flg] -> Logical Operator51/1
  Constant45/1 -> Relational Operator2/2
  Logical Operator51/1 -> Logical Operator48/3
  Logical Operator48/1 -> [VDDM_Shifter1NoComCFSRls_flg]  "VDDM_Shifter1NoComCFSRls_flg"
  [VDDM_Shifter1NoComCFSRls_flg] -> DTC_Couter4/2
  DTC_Couter4/1 -> [VDDM_Shifter1NoComCFS_flg]  "VDDM_Shifter1NoComCFS_flg"
  [VDDM_Shifter1CSErrCFS_flg] -> VDDM_Shifter1CSErrCFS_flg/1
  [VDDM_Shifter1RCErrCFS_flg] -> VDDM_Shifter1RCErrCFS_flg/1
  [VDDM_Shifter1NoComCFS_flg] -> VDDM_Shifter1NoComCFS_flg/1
  Logical Operator28/1 -> Logical Operator36/4
  [VDDM_Shifter1NoComCFS_flg] -> Logical Operator28/1
  Logical Operator6/1 -> Logical Operator22/4
  [VDDM_Shifter1NoComCFS_flg] -> Logical Operator6/1
  VDDM_Shifter1CSErr_flg/1 -> [VDDM_Shifter1CSErr_flg]
  VDDM_Shifter1RCErr_flg/1 -> [VDDM_Shifter1RCErr_flg]
  Switch2/1 -> Test Detection Criteria3/1
  Switch1/1 -> Test Detection Criteria2/1
  Test Detection Criteria3/1 -> [VDDM_Shifter1CSErrDet_flg]  "VDDM_Shifter1CSErrDet_flg"
  [VDDM_Shifter1CSErr_flg] -> Logical Operator26/3
  [DTC_clear_request] -> DTC_Info2/4
  Logical Operator38/1 -> Logical Operator36/3
  Logical Operator26/1 -> Switch2/3
  [VDDM_Shifter1CSErrCFS_flg] -> DTC_Info2/3
  Constant32/1 -> Switch2/1
  [VDDM_Shifter1CSErrCFSRls_flg] -> Switch2/2
  Timer3/1 -> Equal15/1
  Constant41/1 -> Timer3/4
  [task_time_s] -> Test Detection Criteria3/2
  [task_time_s] -> Timer3/3
  [VDDM_Shifter1CSErrDet_flg] -> DTC_Info2/1
  [No_CAN3_BUS_OFF] -> Logical Operator26/2
  [VPMM_SysPwrSta_enum] -> Equal14/1
  DTC_Info2/1 -> VDDM_Shifter1CSErrDTC_raw32/1  "VDDM_Shifter1CSErrDTC_raw32"
  Equal13/1 -> Logical Operator36/1
  [No_CAN3_BUS_OFF] -> Logical Operator36/2
  [VDDM_Shifter1CSErrPass_flg] -> DTC_Info2/2
  Constant35/1 -> Test Detection Criteria3/4
  Constant31/1 -> Equal14/2
  Constant36/1 -> Equal13/2
  [VDDM_Shifter1CSErr_flg] -> Logical Operator38/1
  Constant34/1 -> Equal15/2
  [VDDM_Shifter1NoComCFS_flg] -> Logical Operator34/1
  Logical Operator36/1 -> Logical Operator30/1, Timer3/1
  Equal14/1 -> Logical Operator26/1
  Equal15/1 -> [VDDM_Shifter1CSErrPass_flg]  "VDDM_Shifter1CSErrPass_flg"
  Constant33/1 -> Test Detection Criteria3/3
  [VPMM_SysPwrSta_enum] -> Equal13/1
  Logical Operator30/1 -> Timer3/2
  Logical Operator34/1 -> Logical Operator26/4
  Test Detection Criteria2/1 -> [VDDM_Shifter1RCErrDet_flg]  "VDDM_Shifter1RCErrDet_flg"
  [VDDM_Shifter1RCErr_flg] -> Logical Operator4/3
  [DTC_clear_request] -> DTC_Info1/4
  Logical Operator24/1 -> Logical Operator22/3
  Logical Operator4/1 -> Switch1/3
  [VDDM_Shifter1RCErrCFS_flg] -> DTC_Info1/3
  Constant12/1 -> Switch1/1
  [VDDM_Shifter1RCErrCFSRls_flg] -> Switch1/2
  Timer1/1 -> Equal8/1
  Constant27/1 -> Timer1/4
  [task_time_s] -> Test Detection Criteria2/2
  [task_time_s] -> Timer1/3
  [VDDM_Shifter1RCErrDet_flg] -> DTC_Info1/1
  [No_CAN3_BUS_OFF] -> Logical Operator4/2
  [VPMM_SysPwrSta_enum] -> Equal5/1
  DTC_Info1/1 -> VDDM_Shifter1RCErrDTC_raw32/1  "VDDM_Shifter1RCErrDTC_raw32"
  Equal4/1 -> Logical Operator22/1
  [No_CAN3_BUS_OFF] -> Logical Operator22/2
  [VDDM_Shifter1RCErrPass_flg] -> DTC_Info1/2
  Constant18/1 -> Test Detection Criteria2/4
  Constant11/1 -> Equal5/2
  Constant19/1 -> Equal4/2
  [VDDM_Shifter1RCErr_flg] -> Logical Operator24/1
  Constant14/1 -> Equal8/2
  [VDDM_Shifter1NoComCFS_flg] -> Logical Operator20/1
  Logical Operator22/1 -> Logical Operator12/1, Timer1/1
  Equal5/1 -> Logical Operator4/1
  Equal8/1 -> [VDDM_Shifter1RCErrPass_flg]  "VDDM_Shifter1RCErrPass_flg"
  Constant13/1 -> Test Detection Criteria2/3
  [VPMM_SysPwrSta_enum] -> Equal4/1
  Logical Operator12/1 -> Timer1/2
  Logical Operator20/1 -> Logical Operator4/4
  Constant2/1 -> Switch6/1
  Logical Operator10/1 -> Switch6/3
  Switch6/1 -> Test Detection Criteria1/1
  [VDDM_Shifter1NoComCFSRls_flg] -> Switch6/2
  [DTC_clear_request] -> DTC_Info/4
  No_CAN3_BUS_OFF/1 -> [No_CAN3_BUS_OFF]
  [VDDM_Shifter1NoComDet_flg] -> DTC_Info/1
  DTC_clear_request/1 -> [DTC_clear_request]
  task_time_s/1 -> [task_time_s]
  [VDDM_Shifter1NoComPass_flg] -> DTC_Info/2
  DTC_Info/1 -> VDDM_Shifter1NoComDTC_raw32/1  "VDDM_Shifter1NoComDTC_raw32"
  [VDDM_Shifter1NoComCFS_flg] -> DTC_Info/3
  VPMM_SysPwrSta_enum/1 -> [VPMM_SysPwrSta_enum]
  VDDM_Shifter1NoCom_flg/1 -> [VDDM_Shifter1NoCom_flg]
  [VPMM_SysPwrSta_enum] -> Equal2/1
  [No_CAN3_BUS_OFF] -> Logical Operator7/2
  Constant3/1 -> Equal2/2
  Logical Operator9/1 -> Logical Operator7/3
  Equal2/1 -> Logical Operator7/1
  [VDDM_Shifter1NoCom_flg] -> Logical Operator9/1
  [VPMM_SysPwrSta_enum] -> Equal6/1
  [VDDM_Shifter1NoCom_flg] -> Logical Operator10/3
  Constant17/1 -> Equal6/2
  Equal6/1 -> Logical Operator10/1
  [No_CAN3_BUS_OFF] -> Logical Operator10/2
  [task_time_s] -> Timer2/3
  Constant21/1 -> Equal7/2
  [task_time_s] -> Test Detection Criteria1/2
  Constant70/1 -> Timer2/4
  Constant20/1 -> Test Detection Criteria1/3
  Test Detection Criteria1/1 -> [VDDM_Shifter1NoComDet_flg]  "VDDM_Shifter1NoComDet_flg"
  Equal7/1 -> [VDDM_Shifter1NoComPass_flg]  "VDDM_Shifter1NoComPass_flg"
  Timer2/1 -> Equal7/1
  Logical Operator7/1 -> Timer2/1, Logical Operator14/1
  Constant22/1 -> Test Detection Criteria1/4
  Logical Operator14/1 -> Timer2/2
  [VDDM_Shifter1NoComCFS_flg] -> Logical Operator/1
  [VDDM_Shifter1RCErrCFS_flg] -> Logical Operator/2
  [VDDM_Shifter1CSErrCFS_flg] -> Logical Operator/3
  Logical Operator/1 -> VDDM_Shifter1Err_flg/1  "VDDM_Shifter1Err_flg"
  [VINP_ShifterHandleCmd_enum] -> Equal/1

== system ddm/DDM/DDM/VMC_DDM/ACC Acceleration Command Error ==
  task_time_s : Inport
  VDDM_FCM1NoComCFS_flg : Inport  Port=2
  VDDM_FCM1RCErrCFS_flg : Inport  Port=3
  VDDM_FCM1CSErrCFS_flg : Inport  Port=4
  VVMC_ADASActive_flg : Inport  Port=5
  No_CAN6_BUS_OFF : Inport  Port=6
  VPMM_PowerSta_enum : Inport  Port=7
  VINP_ACCRequireAccel_mps2 : Inport  Port=8
  VINP_ADASACCSta_enum : Inport  Port=9
  DTC_clear_request : Inport  Port=10
  "ACC Acceleration Command Error " : Subsystem
  VDDM_ACCAccelCmdErrCFS_flg : Outport
  VDDM_ACCAccelCmdErrDetDTC_raw32 : Outport  Port=2
  wires:
  [VDDM_ACCAccelCmdErrDetDTC_raw32] -> VDDM_ACCAccelCmdErrDetDTC_raw32/1
  "ACC Acceleration Command Error "/2(VDDM_ACCAccelCmdErrDetDTC_raw32) -> [VDDM_ACCAccelCmdErrDetDTC_raw32]
  VINP_ADASACCSta_enum/1 -> [VINP_ADASACCSta_enum]
  [VINP_ADASACCSta_enum] -> "ACC Acceleration Command Error "/9(VINP_ADASACCSta_enum)
  [VVMC_ADASActive_flg] -> "ACC Acceleration Command Error "/5(VVMC_ADASActive_flg)
  VVMC_ADASActive_flg/1 -> [VVMC_ADASActive_flg]
  [task_time_s] -> "ACC Acceleration Command Error "/1(task_time_s)
  task_time_s/1 -> [task_time_s]  "task_time_s"
  [DTC_clear_request] -> "ACC Acceleration Command Error "/10(DTC_clear_request)
  [VINP_ACCRequireAccel_mps2] -> "ACC Acceleration Command Error "/8(VINP_ACCRequireAccel_mps2)
  [VPMM_PowerSta_enum] -> "ACC Acceleration Command Error "/7(VPMM_PowerSta_enum)
  [No_CAN6_BUS_OFF] -> "ACC Acceleration Command Error "/6(No_CAN6_BUS_OFF)
  [VDDM_FCM1CSErrCFS_flg] -> "ACC Acceleration Command Error "/4(VDDM_FCM1CSErrCFS_flg)
  [VDDM_FCM1RCErrCFS_flg] -> "ACC Acceleration Command Error "/3(VDDM_FCM1RCErrCFS_flg)
  [VDDM_FCM1NoComCFS_flg] -> "ACC Acceleration Command Error "/2(VDDM_FCM1NoComCFS_flg)
  VINP_ACCRequireAccel_mps2/1 -> [VINP_ACCRequireAccel_mps2]
  VDDM_FCM1NoComCFS_flg/1 -> [VDDM_FCM1NoComCFS_flg]
  No_CAN6_BUS_OFF/1 -> [No_CAN6_BUS_OFF]
  VPMM_PowerSta_enum/1 -> [VPMM_PowerSta_enum]
  DTC_clear_request/1 -> [DTC_clear_request]
  "ACC Acceleration Command Error "/1(VDDM_ACCAccelCmdErrCFS_flg) -> [VDDM_ACCAccelCmdErrCFS_flg]
  [VDDM_ACCAccelCmdErrCFS_flg] -> VDDM_ACCAccelCmdErrCFS_flg/1
  VDDM_FCM1RCErrCFS_flg/1 -> [VDDM_FCM1RCErrCFS_flg]
  VDDM_FCM1CSErrCFS_flg/1 -> [VDDM_FCM1CSErrCFS_flg]

== system ddm/DDM/DDM/VMC_DDM/BMS Signal Error  ==
  task_time_s : Inport
  VDDM_C3BMS6LCCFS_flg : Inport  Port=2
  VDDM_C3BMS6RCCFS_flg : Inport  Port=3
  VDDM_C3BMS6CSCFS_flg : Inport  Port=4
  No_CAN3_BUS_OFF : Inport  Port=5
  VPMM_PowerSta_enum : Inport  Port=6
  VINP_BMSWarn8_flg : Inport  Port=7
  VINP_BMSWarn7_flg : Inport  Port=8
  VINP_BMSWarn6_flg : Inport  Port=9
  VINP_BMSWarn5_flg : Inport  Port=10
  VINP_BMSWarn4_flg : Inport  Port=11
  VINP_BMSWarn3_flg : Inport  Port=12
  VINP_BMSWarn2_flg : Inport  Port=13
  VINP_BMSWarn1_flg : Inport  Port=14
  DTC_clear_request : Inport  Port=15
  "BMS Signal Error " : Subsystem
  VDDM_BMSSigErrCFS_flg : Outport
  VDDM_BMSSigErrDetDTC_raw32 : Outport  Port=2
  wires:
  [VDDM_BMSSigErrDetDTC_raw32] -> VDDM_BMSSigErrDetDTC_raw32/1
  "BMS Signal Error "/2(VDDM_BMSSigErrDetDTC_raw32) -> [VDDM_BMSSigErrDetDTC_raw32]
  [task_time_s] -> "BMS Signal Error "/1(task_time_s)
  task_time_s/1 -> [task_time_s]  "task_time_s"
  [VINP_BMSWarn8_flg] -> "BMS Signal Error "/15(VINP_BMSWarn8_flg)
  [VPMM_PowerSta_enum] -> "BMS Signal Error "/6(VPMM_PowerSta_enum)
  [No_CAN3_BUS_OFF] -> "BMS Signal Error "/5(No_CAN3_BUS_OFF)
  [VDDM_C3BMS6RCCFS_flg] -> "BMS Signal Error "/3(VDDM_C3BMS6RCCFS_flg)
  [VDDM_C3BMS6LCCFS_flg] -> "BMS Signal Error "/2(VDDM_C3BMS6LCCFS_flg)
  VINP_BMSWarn4_flg/1 -> [VINP_BMSWarn4_flg]
  VINP_BMSWarn6_flg/1 -> [VINP_BMSWarn6_flg]
  VINP_BMSWarn5_flg/1 -> [VINP_BMSWarn5_flg]
  VINP_BMSWarn7_flg/1 -> [VINP_BMSWarn7_flg]
  VINP_BMSWarn8_flg/1 -> [VINP_BMSWarn8_flg]
  VDDM_C3BMS6LCCFS_flg/1 -> [VDDM_C3BMS6LCCFS_flg]
  No_CAN3_BUS_OFF/1 -> [No_CAN3_BUS_OFF]
  VPMM_PowerSta_enum/1 -> [VPMM_PowerSta_enum]
  DTC_clear_request/1 -> [DTC_clear_request]
  "BMS Signal Error "/1(VDDM_BMSSigErrCFS_flg) -> [VDDM_BMSSigErrCFS_flg]
  [VDDM_BMSSigErrCFS_flg] -> VDDM_BMSSigErrCFS_flg/1
  VDDM_C3BMS6RCCFS_flg/1 -> [VDDM_C3BMS6RCCFS_flg]
  VDDM_C3BMS6CSCFS_flg/1 -> [VDDM_C3BMS6CSCFS_flg]
  [VDDM_C3BMS6CSCFS_flg] -> "BMS Signal Error "/4(VDDM_C3BMS6CSCFS_flg)
  [DTC_clear_request] -> "BMS Signal Error "/10(DTC_clear_request)
  [VINP_BMSWarn5_flg] -> "BMS Signal Error "/12(VINP_BMSWarn5_flg)
  [VINP_BMSWarn4_flg] -> "BMS Signal Error "/11(VINP_BMSWarn4_flg)
  [VINP_BMSWarn6_flg] -> "BMS Signal Error "/13(VINP_BMSWarn6_flg)
  [VINP_BMSWarn7_flg] -> "BMS Signal Error "/14(VINP_BMSWarn7_flg)
  [VINP_BMSWarn1_flg] -> "BMS Signal Error "/7(VINP_BMSWarn1_flg)
  [VINP_BMSWarn2_flg] -> "BMS Signal Error "/8(VINP_BMSWarn2_flg)
  [VINP_BMSWarn3_flg] -> "BMS Signal Error "/9(VINP_BMSWarn3_flg)
  VINP_BMSWarn3_flg/1 -> [VINP_BMSWarn3_flg]
  VINP_BMSWarn2_flg/1 -> [VINP_BMSWarn2_flg]
  VINP_BMSWarn1_flg/1 -> [VINP_BMSWarn1_flg]

== system ddm/DDM/DDM/VMC_DDM/CCU Signal Error ==
  task_time_s : Inport
  VDDM_C3CCU2LCCFS_flg : Inport  Port=2
  VDDM_C3CCU2RCCFS_flg : Inport  Port=3
  VDDM_C3CCU2CSCFS_flg : Inport  Port=4
  No_CAN3_BUS_OFF : Inport  Port=5
  VPMM_PowerSta_enum : Inport  Port=6
  VINP_DCDCFaultSta_enum : Inport  Port=7
  DTC_clear_request : Inport  Port=8
  "CCU Signal Error " : Subsystem
  VDDM_CCUSigErrCFS_flg : Outport
  VDDM_CCUSigErrDetDTC_raw32 : Outport  Port=2
  wires:
  [VDDM_CCUSigErrDetDTC_raw32] -> VDDM_CCUSigErrDetDTC_raw32/1
  "CCU Signal Error "/2(VDDM_CCUSigErrDetDTC_raw32) -> [VDDM_CCUSigErrDetDTC_raw32]
  [task_time_s] -> "CCU Signal Error "/1(task_time_s)
  task_time_s/1 -> [task_time_s]  "task_time_s"
  [DTC_clear_request] -> "CCU Signal Error "/8(DTC_clear_request)
  [VINP_DCDCFaultSta_enum] -> "CCU Signal Error "/7(VINP_DCDCFaultSta_enum)
  [VPMM_PowerSta_enum] -> "CCU Signal Error "/6(VPMM_PowerSta_enum)
  [No_CAN3_BUS_OFF] -> "CCU Signal Error "/5(No_CAN3_BUS_OFF)
  [VDDM_C3CCU2CSCFS_flg] -> "CCU Signal Error "/4(VDDM_C3CCU2CSCFS_flg)
  [VDDM_C3CCU2RCCFS_flg] -> "CCU Signal Error "/3(VDDM_C3CCU2RCCFS_flg)
  [VDDM_C3CCU2LCCFS_flg] -> "CCU Signal Error "/2(VDDM_C3CCU2LCCFS_flg)
  VINP_DCDCFaultSta_enum/1 -> [VINP_DCDCFaultSta_enum]
  VDDM_C3CCU2LCCFS_flg/1 -> [VDDM_C3CCU2LCCFS_flg]
  No_CAN3_BUS_OFF/1 -> [No_CAN3_BUS_OFF]
  VPMM_PowerSta_enum/1 -> [VPMM_PowerSta_enum]
  DTC_clear_request/1 -> [DTC_clear_request]
  "CCU Signal Error "/1(VDDM_CCUSigErrCFS_flg) -> [VDDM_CCUSigErrCFS_flg]
  [VDDM_CCUSigErrCFS_flg] -> VDDM_CCUSigErrCFS_flg/1
  VDDM_C3CCU2RCCFS_flg/1 -> [VDDM_C3CCU2RCCFS_flg]
  VDDM_C3CCU2CSCFS_flg/1 -> [VDDM_C3CCU2CSCFS_flg]

== system ddm/DDM/DDM/VMC_DDM/ESC Signal Error ==
  task_time_s : Inport
  No_CAN1_BUS_OFF : Inport  Port=2
  VPMM_PowerSta_enum : Inport  Port=3
  DTC_clear_request : Inport  Port=4
  VINP_ABSFailed_flg : Inport  Port=5
  VINP_TCSFailed_flg : Inport  Port=6
  VINP_ESCFailed_flg : Inport  Port=7
  VINP_HSAFailed_flg : Inport  Port=8
  VINP_AVHFailed_flg : Inport  Port=9
  VINP_MCPressureV_flg : Inport  Port=10
  VINP_BrkSwV_flg : Inport  Port=11
  VINP_BrkPedalPosSta_flg : Inport  Port=12
  VINP_LongAccelV_flg : Inport  Port=13
  VINP_LatAccelV_flg : Inport  Port=14
  VINP_YawRateV_flg : Inport  Port=15
  VINP_LRRawWhlSpeedV_flg : Inport  Port=16
  VINP_RRRawWhlSpeedV_flg : Inport  Port=17
  VINP_LFRawWhlSpeedV_flg : Inport  Port=18
  VINP_RFRawWhlSpeedV_flg : Inport  Port=19
  VINP_VehSpeed_kph : Inport  Port=20
  VINP_FrntAxlTrqReqDrv_Nm : Inport  Port=21
  VINP_RearAxlTrqReqDrv_Nm : Inport  Port=22
  VDDM_ESC1Err_flg : Inport  Port=23
  VDDM_ESC5Err_flg : Inport  Port=24
  VINP_GRADE_Deg : Inport  Port=25
  VINP_FrntAxlTrqReqBrk_Nm : Inport  Port=26
  VINP_RearAxlTrqReqBrk_Nm : Inport  Port=27
  VINP_ESCAPSSta_enum : Inport  Port=28
  "ESC Signal Error " : Subsystem
  VDDM_ESCSigErrCFS_flg : Outport
  VDDM_ESCSigErrDetDTC_raw32 : Outport  Port=2
  VDDM_ESC1SigErr_flg : Outport  Port=3
  VDDM_ESC5SigErr_flg : Outport  Port=4
  wires:
  [VDDM_ESC5SigErr_flg] -> VDDM_ESC5SigErr_flg/1
  [VDDM_ESC1SigErr_flg] -> VDDM_ESC1SigErr_flg/1
  "ESC Signal Error "/4(VDDM_ESC5SigErr_flg) -> [VDDM_ESC5SigErr_flg]
  "ESC Signal Error "/3(VDDM_ESC1SigErr_flg) -> [VDDM_ESC1SigErr_flg]
  [VINP_RFRawWhlSpeedV_flg] -> "ESC Signal Error "/19(VINP_RFRawWhlSpeedV_flg)
  [VINP_LFRawWhlSpeedV_flg] -> "ESC Signal Error "/18(VINP_LFRawWhlSpeedV_flg)
  [VINP_RRRawWhlSpeedV_flg] -> "ESC Signal Error "/17(VINP_RRRawWhlSpeedV_flg)
  [VINP_LRRawWhlSpeedV_flg] -> "ESC Signal Error "/16(VINP_LRRawWhlSpeedV_flg)
  VINP_RFRawWhlSpeedV_flg/1 -> [VINP_RFRawWhlSpeedV_flg]
  VINP_RRRawWhlSpeedV_flg/1 -> [VINP_RRRawWhlSpeedV_flg]
  VINP_LFRawWhlSpeedV_flg/1 -> [VINP_LFRawWhlSpeedV_flg]
  VINP_LRRawWhlSpeedV_flg/1 -> [VINP_LRRawWhlSpeedV_flg]
  [VDDM_ESCSigErrCFS_flg] -> VDDM_ESCSigErrCFS_flg/1
  [VINP_YawRateV_flg] -> "ESC Signal Error "/15(VINP_YawRateV_flg)
  [VINP_LatAccelV_flg] -> "ESC Signal Error "/14(VINP_LatAccelV_flg)
  [VINP_LongAccelV_flg] -> "ESC Signal Error "/13(VINP_LongAccelV_flg)
  [VINP_BrkPedalPosSta_flg] -> "ESC Signal Error "/12(VINP_BrkPedalPosSta_flg)
  [VINP_BrkSwV_flg] -> "ESC Signal Error "/11(VINP_BrkSwV_flg)
  [VINP_MCPressureV_flg] -> "ESC Signal Error "/10(VINP_MCPressureV_flg)
  [VINP_AVHFailed_flg] -> "ESC Signal Error "/9(VINP_AVHFailed_flg)
  [VINP_HSAFailed_flg] -> "ESC Signal Error "/8(VINP_HSAFailed_flg)
  [VINP_ESCFailed_flg] -> "ESC Signal Error "/7(VINP_ESCFailed_flg)
  [VINP_TCSFailed_flg] -> "ESC Signal Error "/6(VINP_TCSFailed_flg)
  [VINP_ABSFailed_flg] -> "ESC Signal Error "/5(VINP_ABSFailed_flg)
  VINP_YawRateV_flg/1 -> [VINP_YawRateV_flg]
  VINP_LatAccelV_flg/1 -> [VINP_LatAccelV_flg]
  VINP_LongAccelV_flg/1 -> [VINP_LongAccelV_flg]
  VINP_BrkPedalPosSta_flg/1 -> [VINP_BrkPedalPosSta_flg]
  VINP_BrkSwV_flg/1 -> [VINP_BrkSwV_flg]
  VINP_MCPressureV_flg/1 -> [VINP_MCPressureV_flg]
  VINP_AVHFailed_flg/1 -> [VINP_AVHFailed_flg]
  VINP_HSAFailed_flg/1 -> [VINP_HSAFailed_flg]
  VINP_ESCFailed_flg/1 -> [VINP_ESCFailed_flg]
  VINP_TCSFailed_flg/1 -> [VINP_TCSFailed_flg]
  VINP_ABSFailed_flg/1 -> [VINP_ABSFailed_flg]
  "ESC Signal Error "/1(VDDM_ESCSigErrCFS_flg) -> [VDDM_ESCSigErrCFS_flg]
  DTC_clear_request/1 -> [DTC_clear_request]
  VPMM_PowerSta_enum/1 -> [VPMM_PowerSta_enum]
  No_CAN1_BUS_OFF/1 -> [No_CAN1_BUS_OFF]
  [No_CAN1_BUS_OFF] -> "ESC Signal Error "/2(No_CAN1_BUS_OFF)
  [VPMM_PowerSta_enum] -> "ESC Signal Error "/3(VPMM_PowerSta_enum)
  [DTC_clear_request] -> "ESC Signal Error "/4(DTC_clear_request)
  task_time_s/1 -> [task_time_s]  "task_time_s"
  [task_time_s] -> "ESC Signal Error "/1(task_time_s)
  "ESC Signal Error "/2(VDDM_ESCSigErrDetDTC_raw32) -> [VDDM_ESCSigErrDetDTC_raw32]
  [VDDM_ESCSigErrDetDTC_raw32] -> VDDM_ESCSigErrDetDTC_raw32/1
  [VINP_VehSpeed_kph] -> "ESC Signal Error "/20(VINP_VehSpeed_kph)
  [VINP_FrntAxlTrqReqDrv_Nm] -> "ESC Signal Error "/21(VINP_FrntAxlTrqReqDrv_Nm)
  [VINP_RearAxlTrqReqDrv_Nm] -> "ESC Signal Error "/22(VINP_RearAxlTrqReqDrv_Nm)
  [VDDM_ESC1Err_flg] -> "ESC Signal Error "/23(VDDM_ESC1Err_flg)
  [VDDM_ESC5Err_flg] -> "ESC Signal Error "/24(VDDM_ESC5Err_flg)
  [VINP_GRADE_Deg] -> "ESC Signal Error "/25(VINP_GRADE_Deg)
  [VINP_FrntAxlTrqReqBrk_Nm] -> "ESC Signal Error "/26(VINP_FrntAxlTrqReqBrk_Nm)
  [VINP_RearAxlTrqReqBrk_Nm] -> "ESC Signal Error "/27(VINP_RearAxlTrqReqBrk_Nm)
  [VINP_ESCAPSSta_enum] -> "ESC Signal Error "/28(VINP_ESCAPSSta_enum)
  VINP_VehSpeed_kph/1 -> [VINP_VehSpeed_kph]
  VINP_FrntAxlTrqReqBrk_Nm/1 -> [VINP_FrntAxlTrqReqBrk_Nm]
  VDDM_ESC1Err_flg/1 -> [VDDM_ESC1Err_flg]
  VINP_RearAxlTrqReqBrk_Nm/1 -> [VINP_RearAxlTrqReqBrk_Nm]
  VINP_GRADE_Deg/1 -> [VINP_GRADE_Deg]
  VDDM_ESC5Err_flg/1 -> [VDDM_ESC5Err_flg]
  VINP_FrntAxlTrqReqDrv_Nm/1 -> [VINP_FrntAxlTrqReqDrv_Nm]
  VINP_RearAxlTrqReqDrv_Nm/1 -> [VINP_RearAxlTrqReqDrv_Nm]
  VINP_ESCAPSSta_enum/1 -> [VINP_ESCAPSSta_enum]
